simulink model "FuzzyModel"  (R2020a)
settings: Solver=VariableStepAuto  StartTime=0.0  StopTime=10.0  RelTol=1e-3
values from neighbouring files (symbols this model uses):
  dijastolniPritisak = str2num(get(handles.edit2,'string'))    [GUI.m]
  glukoza = str2num(get(handles.edit4,'string'))    [GUI.m]
  hdlc = str2num(get(handles.edit6,'string'))    [GUI.m]
  obimStruka = str2num(get(handles.edit1,'string'))    [GUI.m]
  sistolniPritisak = str2num(get(handles.edit3,'string'))    [GUI.m]
  trigliceridi = str2num(get(handles.edit5,'string'))    [GUI.m]
libraries: neural x255, fuzblock x1
(part 4 of 4)

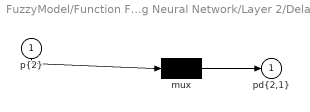
== system FuzzyModel/Function Fitting Neural Network/Layer 2/Delays 1 ==
  "p{2}" : Inport  PortDimensions=250
      mask Display: e = 0.06;c1 = [120 230 180]/255;c2 = ([120 230 180]+0)/(256+128);c3 = ([120 230 180]+128)/(256+128);patch([0 1 1 0],[0 0 1 1],c1);patch([0 1 1 1-e 1-e 0+e],[0 0 1 1-e 0+e 0+e],c2);patch([0 0 1 1-e 0+e 0+e],[0 1 1 1-e 1-e 0+e],c3);plot([0 1 1 0 0],[0 0 1 1 0]);
  mux : Mux  Inputs=1
      mask Display: e = 0.06;c1 = [120 150 230]/255;c2 = ([120 150 230]+0)/383;c3 = ([120 150 230]+128)/383;patch([0 1 1 0],[0 0 1 1],c1);patch([0 1 1 1-e 1-e 0+e],[0 0 1 1-e 0+e 0+e],c2);patch([0 0 1 1-e 0+e 0+e],[0 1 1 1-e 1-e 0+e],c3);plot([0 1 1 0 0],[0 0 1 1 0]);disp('Mux')
  "pd{2,1}" : Outport
      mask Display: e = 0.06;c1 = [120 230 180]/255;c2 = ([120 230 180]+0)/(256+128);c3 = ([120 230 180]+128)/(256+128);patch([0 1 1 0],[0 0 1 1],c1);patch([0 1 1 1-e 1-e 0+e],[0 0 1 1-e 0+e 0+e],c2);patch([0 0 1 1-e 0+e 0+e],[0 1 1 1-e 1-e 0+e],c3);plot([0 1 1 0 0],[0 0 1 1 0]);
  wires:
  "p{2}"/1 -> mux/1
  mux/1 -> "pd{2,1}"/1

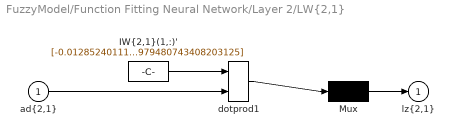
== system FuzzyModel/Function Fitting Neural Network/Layer 2/LW{2,1} ==
  "ad{2,1}" : Inport  PortDimensions=250
      mask Display: e = 0.06;c1 = [120 230 180]/255;c2 = ([120 230 180]+0)/(256+128);c3 = ([120 230 180]+128)/(256+128);patch([0 1 1 0],[0 0 1 1],c1);patch([0 1 1 1-e 1-e 0+e],[0 0 1 1-e 0+e 0+e],c2);patch([0 0 1 1-e 0+e 0+e],[0 1 1 1-e 1-e 0+e],c3);plot([0 1 1 0 0],[0 0 1 1 0]);
  "IW{2,1}(1,:)'" : Constant  Value=[-0.012852401115615370852385268563011777587234973907470703125;0.02934266499093089730632044620506349019706249237060546875;0.01264020343172586428870385333311787690035998821258544921875;-0.0579423951830408678898010066404822282493114471435546875;0.0179405340234247805131229114294910687021911144256591796875;-0.01136069133129583887120706009454806917347013950347900390625;-0.002968864774904622118312236267456682980991899967193603515625;0.16263779143132184312747767762630246579647064208984375;0.0246135774386968368687700348118596593849360942840576171875;-0.020403349455339177265233985281156492419540882110595703125;0.009482358206311415627087768598357797600328922271728515625;-0.14000087101994151961292800478986464440822601318359375;0.010399833527627098950230077889500535093247890472412109375;-0.330321959610481885594168716124841012060642242431640625;0.262613373850480613658220363504369743168354034423828125;0.027021189362813870238344549079556600190699100494384765625;-0.001169795675316554796341339539367254474200308322906494140625;0.0239316030987301690824420319358978304080665111541748046875;-0.0258641924884518183136439262170824804343283176422119140625;-0.00511340793857374513453617481673063593916594982147216796875;0.0178564557933434155112539798437865101732313632965087890625;-0.00931754704092221074096524802143903798423707485198974609375;0.002318596003681310489807909647197448066435754299163818359375;-0.074703795729715249951397026961785741150379180908203125;-0.00280225803370762020783057977268981630913913249969482421875;0.01166688355577617797198541893521905876696109771728515625;-0.005060820406904872371944836828561165020801126956939697265625;-0.1316086810196624157232037077847053296864032745361328125;-0.0183116048229094129096150567193035385571420192718505859375;0.0424925515296023237343803202747949399054050445556640625;0.0147088547085950267778731159751259838230907917022705078125;0.000151340925825352496693343429257083698757924139499664306640625;0.004708579495979203950739577777540034730918705463409423828125;0.03429379588128030065252715985479881055653095245361328125;-0.0032412335264143314443596732843388963374309241771697998046875;0.02364422510538700950011303802966722287237644195556640625;0.0175535660663491965838289843304664827883243560791015625;0.0080458874237034870569029720854814513586461544036865234375;0.0073575627713586000400169950808049179613590240478515625;-0.0190769135495804549595977306353233871050179004669189453125;0.0170264130183285684883021104951694724150002002716064453125;-0.023714474399154576722548171119342441670596599578857421875;-0.01389723486316142390950556517736913519911468029022216796875;-0.0003641890436542306809693247959813788838800974190235137939453125;0.023363991355441156294592275344257359392940998077392578125;-0.0110508928287409123603080018938271678052842617034912109375;-0.01215803619675769053909419881165376864373683929443359375;-0.01536545932332272247633486728091156692244112491607666015625;0.000957938068568726301503513109736331898602657020092010498046875;0.00105515037816005137483177378499021870084106922149658203125;0.01191012660951402436781965121781468042172491550445556640625;0.009062829977406393344718793514402932487428188323974609375;0.000384428105878272647309701337547949151485227048397064208984375;-0.00932169850448842131351856465926175587810575962066650390625;-0.0258523040145362988095900647067537647671997547149658203125;-0.0111881724176340520415795509734380175359547138214111328125;0.005093564520564537734248489186938968487083911895751953125;-0.005206585210700325795640797110763742239214479923248291015625;0.0023951824751550217056095259948733655619435012340545654296875;-0.0078043634939143104178871368503678240813314914703369140625;0.0078417596303808588531492063111727475188672542572021484375;0.666892512875574272612766435486264526844024658203125;-0.001036419918916799652597315883895134902559220790863037109375;-0.0244897161567864292408547299828569521196186542510986328125;-0.015734174570663915504464824834940372966229915618896484375 ...(+11354 chars)]
      mask Display: e = 0.06;c1 = [120 150 230]/255;c2 = ([120 150 230]+0)/383;c3 = ([120 150 230]+128)/383;patch([0 1 1 0],[0 0 1 1],c1);patch([0 1 1 1-e 1-e 0+e],[0 0 1 1-e 0+e 0+e],c2);patch([0 0 1 1-e 0+e 0+e],[0 1 1 1-e 1-e 0+e],c3);plot([0 1 1 0 0],[0 0 1 1 0]);disp('weights');
  Mux : Mux  Inputs=1
      mask Display: e = 0.06;c1 = [120 150 230]/255;c2 = ([120 150 230]+0)/383;c3 = ([120 150 230]+128)/383;patch([0 1 1 0],[0 0 1 1],c1);patch([0 1 1 1-e 1-e 0+e],[0 0 1 1-e 0+e 0+e],c2);patch([0 0 1 1-e 0+e 0+e],[0 1 1 1-e 1-e 0+e],c3);plot([0 1 1 0 0],[0 0 1 1 0]);disp('Mux');
  dotprod1 : neural/Weight Functions/dotprod
  "lz{2,1}" : Outport
      mask Display: e = 0.06;c1 = [120 230 180]/255;c2 = ([120 230 180]+0)/(256+128);c3 = ([120 230 180]+128)/(256+128);patch([0 1 1 0],[0 0 1 1],c1);patch([0 1 1 1-e 1-e 0+e],[0 0 1 1-e 0+e 0+e],c2);patch([0 0 1 1-e 0+e 0+e],[0 1 1 1-e 1-e 0+e],c3);plot([0 1 1 0 0],[0 0 1 1 0]);
  wires:
  "IW{2,1}(1,:)'"/1 -> dotprod1/1
  "ad{2,1}"/1 -> dotprod1/2
  dotprod1/1 -> Mux/1
  Mux/1 -> "lz{2,1}"/1
